simulink model "untuk_SS_closedLoop"  (R2021b)
settings: Solver=VariableStepAuto  StartTime=0.0  StopTime=1680  RelTol=1e-3
undefined symbols (not defined in the file): alpha, lr_init, selectorSP, sigbuilder_block, SP
libraries: slpidlib x1
settings Model: Creator=Asus  LastModifiedBy=Asus

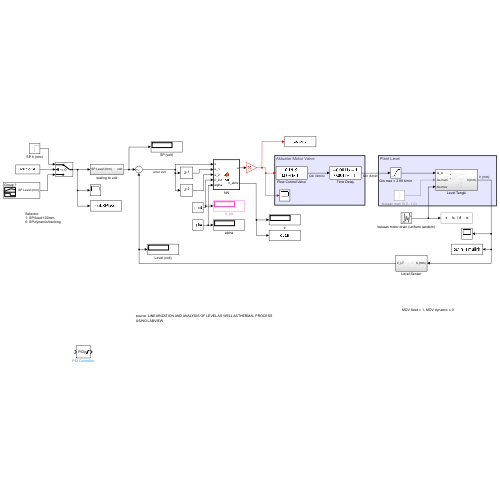
[thumbnail: Simulink's stored preview of the top-level diagram]
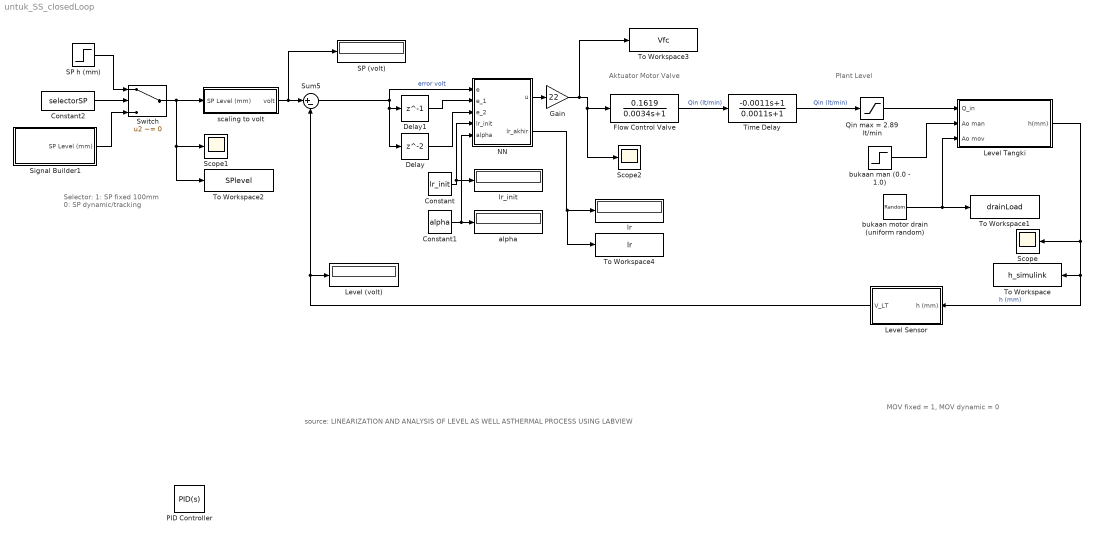
== system untuk_SS_closedLoop ==
  note: Selector:
      | 1: SP fixed 100mm
      | 0: SP dynamic/tracking
  note: Aktuator Motor Valve
  note: Plant Level
  note: source: LINEARIZATION AND ANALYSIS OF LEVEL AS WELL ASTHERMAL PROCESS USING LABVIEW
  note: MOV fixed = 1, MOV dynamic = 0
  Constant : Constant  Value=lr_init
  Constant1 : Constant  Value=alpha
  Constant2 : Constant  Value=selectorSP
  Delay : Delay  InitialCondition=0
  Delay1 : Delay  DelayLength=1  InitialCondition=0
  Flow Control Valve : TransferFcn  Numerator=[0.1619]  Denominator=[0.0034 1]
  Gain : Gain  Gain=22
  Level (volt) : Display
  Level Sensor : Subsystem
  Level Tangki : Subsystem
  NN : MATLAB Function  TreatAsAtomicUnit=on
  PID Controller : slpidlib/PID Controller  Controller=PID  Form=Parallel  TimeDomain=Continuous-time  UseExternalTs=off  SampleTime=-1  IntegratorMethod=Forward Euler  FilterMethod=Forward Euler  ControllerParametersSource=internal  P=13.8  I=0.256  D=0  UseFilter=on  N=100  TunerSelectOption=Transfer Function Based (PID Tuner App)  InitialConditionSource=internal  InitialConditionForIntegrator=0  InitialConditionForFilter=0  DifferentiatorICPrevScaledInput=0  ExternalReset=none  TrackingMode=off  Kt=1  LimitOutput=on  SatLimitsSource=internal  UpperSaturationLimit=22  LowerSaturationLimit=0  LinearizeAsGain=on  AntiWindupMode=none  Kb=1  POutMin=[]  POutMax=[]  IOutMin=[]  IOutMax=[]  DOutMin=[]  DOutMax=[]  NOutMin=[]  NOutMax=[]  SumOutMin=[]  SumOutMax=[]  SaturationOutMin=[]  SaturationOutMax=[]  PParamMin=[]  PParamMax=[]  IParamMin=[]  IParamMax=[]  DParamMin=[]  DParamMax=[]  NParamMin=[]  NParamMax=[]  KbParamMin=[]  KbParamMax=[]  KtParamMin=[]  KtParamMax=[]  KbOutMin=[]  KbOutMax=[]  KtOutMin=[]  KtOutMax=[]  IntegratorOutMin=[]  IntegratorOutMax=[]  FilterOutMin=[]  FilterOutMax=[]  SumI1OutMin=[]  SumI1OutMax=[]  SumI2OutMin=[]  SumI2OutMax=[]  SumI3OutMin=[]  SumI3OutMax=[]  SumI4OutMin=[]  SumI4OutMax=[]  SumDOutMin=[]  SumDOutMax=[]  DifferentiatorOutMin=[]  DifferentiatorOutMax=[]  FilterDiffOutCoefMin=[]  FilterDiffOutCoefMax=[]  ReciprocalOutMin=[]  ReciprocalOutMax=[]  SumDenOutMin=[]  SumDenOutMax=[]  SumNumOutMin=[]  SumNumOutMax=[]  DivideOutMin=[]  DivideOutMax=[]  UdiffTsProdOutMin=[]  UdiffTsProdOutMax=[]  NTsProdOutMin=[]  NTsProdOutMax=[]  UintegralTsProdOutMin=[]  UintegralTsProdOutMax=[]  UngainTsProdOutMin=[]  UngainTsProdOutMax=[]  IntegratorContinuousStateAttributes=''  IntegratorStateMustResolveToSignalObject=off  IntegratorRTWStateStorageClass=Auto  FilterContinuousStateAttributes=''  FilterStateMustResolveToSignalObject=off  FilterRTWStateStorageClass=Auto  ParallelPVariant=InternalParameters  IdealPVariant=Disabled  IVariant=InternalParameters  DVariant=InternalParameters  IntegratorVariant=Continuous  SatVariant=Enabled  AWVariant=Passthrough  PCopyVariant=Disabled  TRVariant=Disabled  FdbkBlocksVariant=Forward  IdealPFdbkVariant=Disabled  SatFdbkVariant=Disabled  DerivativeFilterVariant=ContFilter  NVariant=InternalParameters  NCopyVariant=Disabled  FilterICVariant=InternalICsFilter  IntegratorICVariant=InternalICs  ExternalResetVariant=Disabled  TRSumVariant=Passthrough  SumFdbkVariant=Disabled  SumVariant=Sum_PID  TsampFilterVariant=InternalTs  TsampNgainVariant=Passthrough  TsampIntegralVariant=Passthrough  ExternalSaturationOutDataTypeStr=Inherit: Same as second input
  Qin max = 2.89 lt/min : Saturate  UpperLimit=2.89254556517870  LowerLimit=0
  SP (volt) : Display
  SP h (mm) : Step  Time=0  After=SP  SampleTime=0.1
  Scope : Scope
  Scope1 : Scope
  Scope2 : Scope
  Signal Builder1 : Subsystem  Tag=STV Subsys  LoadFcn=sigbuilder_block('load');  StartFcn=sigbuilder_block('start');  StopFcn=sigbuilder_block('stop');  ClipboardFcn=sigbuilder_block('clipboard');  mask(Sigbuilder block){tuvar=[0:10]}
      mask help: Simulink:masks:SigbuilderBlock_MD
      mask init:
      | if ~strcmp(get_param(bdroot(gcbh),'SimulationStatus'),'stopped') tuvar = sigbuilder_block('maskInit'); end
      settings: CopyFcn=sigbuilder_block('copy');  DeleteFcn=sigbuilder_block('delete');  ModelCloseFcn=sigbuilder_block('modelClose');  PreSaveFcn=sigbuilder_block('preSave');  PauseFcn=sigbuilder_block('pause');  ContinueFcn=sigbuilder_block('continue');  NameChangeFcn=sigbuilder_block('namechange');  OpenFcn=sigbuilder_block('open',[572.4 148.2 550.8 400.2 ]);  CloseFcn=sigbuilder_block('close');
      mask Display: plot(0, 0, 100, 100,[2, 2, 32, 32, 2], [68, 8, 8, 68, 68],[32, 2], [38, 38], [32, 19, 2],[53, 60, 44], [32, 17, 17, 2],[16, 16, 31, 31]);txt = getActiveGroup(gcbh);text(2, 100, txt,'verticalAlignment', 'top');
  Sum5 : Sum  Inputs=|+-
  Switch : Switch  Criteria=u2 ~= 0
  Time Delay : TransferFcn  Numerator=[-0.0011 1]  Denominator=[0.0011 1]
  To Workspace : ToWorkspace  VariableName=h_simulink  SampleTime=-1
      settings: Save2DSignal=2-D array (concatenate along first dimension)
  To Workspace1 : ToWorkspace  VariableName=drainLoad  SampleTime=-1
  To Workspace2 : ToWorkspace  VariableName=SPlevel  SampleTime=-1
  To Workspace3 : ToWorkspace  VariableName=Vfc  SampleTime=-1
  To Workspace4 : ToWorkspace  VariableName=lr  SampleTime=-1
  alpha : Display
  bukaan man (0.0 - 1.0) : Step  Time=0  SampleTime=0
  bukaan motor drain (uniform random) : UniformRandomNumber  Minimum=0  SampleTime=15
  lr : Display
  lr_init : Display
  scaling to volt : Subsystem
  wires:
  Sum5/1 -> Delay/1, Delay1/1, NN/1(e)  "error volt"
  Delay1/1 -> NN/2(e_1)
  Delay/1 -> NN/3(e_2)
  Level Tangki/1(h(mm)) -> Level Sensor/1(h (mm)), To Workspace/1, Scope/1  "h (mm)"
  Qin max = 2.89 lt/min/1 -> Level Tangki/1(Q_in)
  Level Sensor/1(V_LT) -> Sum5/2, Level (volt)/1
  bukaan man (0.0 - 1.0)/1 -> Level Tangki/2(Ao man)
  bukaan motor drain (uniform random)/1 -> Level Tangki/3(Ao mov), To Workspace1/1
  scaling to volt/1(volt) -> SP (volt)/1, Sum5/1
  Switch/1 -> scaling to volt/1(SP Level (mm)), To Workspace2/1, Scope1/1
  Constant/1 -> NN/4(lr_init), lr_init/1
  Constant1/1 -> NN/5(alpha), alpha/1
  SP h (mm)/1 -> Switch/1
  Signal Builder1/1(SP Level (mm)) -> Switch/3
  Constant2/1 -> Switch/2
  NN/2(lr_akhir) -> To Workspace4/1, lr/1
  Flow Control Valve/1 -> Time Delay/1  "Qin (lt/min)"
  Time Delay/1 -> Qin max = 2.89 lt/min/1  "Qin (lt/min)"
  Gain/1 -> To Workspace3/1, Scope2/1, Flow Control Valve/1
  NN/1(u) -> Gain/1

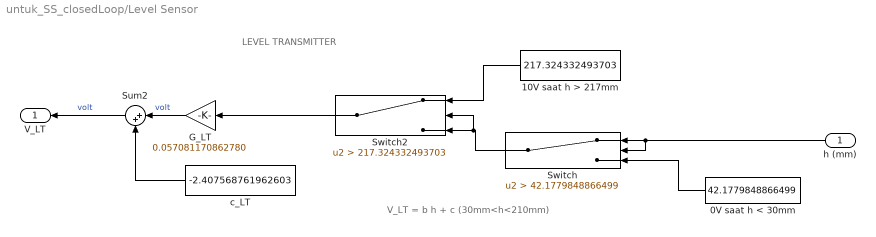
== system untuk_SS_closedLoop/Level Sensor ==
  note: V_LT = b h + c (30mm<h<210mm)
  note: LEVEL TRANSMITTER
  h (mm) : Inport
  0V saat h < 30mm : Constant  Value=42.1779848866499
  10V saat h > 217mm : Constant  Value=217.324332493703
  G_LT : Gain  Gain=0.057081170862780
  Sum2 : Sum  Inputs=|++
  Switch : Switch  Criteria=u2 > Threshold  Threshold=42.1779848866499
  Switch2 : Switch  Criteria=u2 > Threshold  Threshold=217.324332493703
  c_LT : Constant  Value=-2.407568761962603
  V_LT : Outport
  wires:
  Switch/1 -> Switch2/2, Switch2/3
  10V saat h > 217mm/1 -> Switch2/1
  G_LT/1 -> Sum2/1  "volt"
  0V saat h < 30mm/1 -> Switch/3
  c_LT/1 -> Sum2/2
  h (mm)/1 -> Switch/2, Switch/1
  Switch2/1 -> G_LT/1
  Sum2/1 -> V_LT/1  "volt"

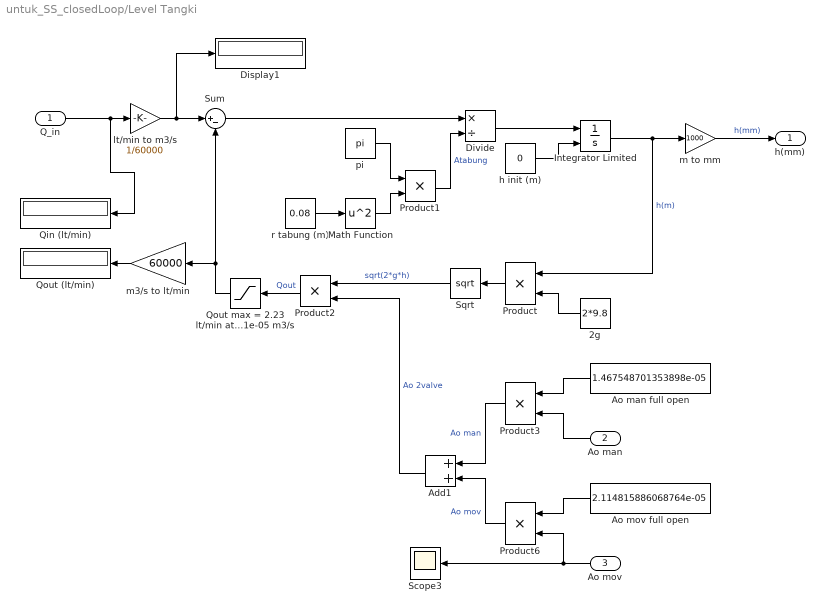
== system untuk_SS_closedLoop/Level Tangki ==
  Q_in : Inport
  Ao man : Inport  Port=2
  Ao mov : Inport  Port=3
  2g : Constant  Value=2*9.8
  Add1 : Sum
  Ao man full open : Constant  Value=1.467548701353898e-05
  Ao mov full open : Constant  Value=2.114815886068764e-05
  Display1 : Display
  Divide : Product  Inputs=*/
  Integrator Limited : Integrator  InitialConditionSource=external  LimitOutput=on  UpperSaturationLimit=1  LowerSaturationLimit=0
  Math Function : Math  Operator=square  SaturateOnIntegerOverflow=on
  Product{,1..3,6} (5 alike) : Product
  Qin (lt/min) : Display
  Qout (lt/min) : Display
  Qout max = 2.23 lt/min atau 3.716859357396591e-05 m3/s : Saturate  UpperLimit=3.716859357396591e-05  LowerLimit=0
  Scope3 : Scope
  Sqrt : Sqrt  SaturateOnIntegerOverflow=on
  Sum : Sum  Inputs=|+-
  h init (m) : Constant  Value=0
  lt/min to m3/s : Gain  Gain=1/60000
  m to mm : Gain  Gain=1000
  m3/s to lt/min : Gain  Gain=60000
  pi : Constant  Value=pi
  r tabung (m) : Constant  Value=0.08
  h(mm) : Outport
  wires:
  Sqrt/1 -> Product2/1  "sqrt(2*g*h)"
  h init (m)/1 -> Integrator Limited/2
  Sum/1 -> Divide/1
  Math Function/1 -> Product1/2
  Qout max = 2.23 lt/min atau 3.716859357396591e-05 m3/s/1 -> Sum/2, m3/s to lt/min/1
  Integrator Limited/1 -> Product/1, m to mm/1  "h(m)"
  Divide/1 -> Integrator Limited/1
  r tabung (m)/1 -> Math Function/1
  Product1/1 -> Divide/2  "Atabung"
  lt/min to m3/s/1 -> Display1/1, Sum/1
  pi/1 -> Product1/1
  Product/1 -> Sqrt/1
  m3/s to lt/min/1 -> Qout (lt/min)/1
  Q_in/1 -> Qin (lt/min)/1, lt/min to m3/s/1
  Product2/1 -> Qout max = 2.23 lt/min atau 3.716859357396591e-05 m3/s/1  "Qout"
  2g/1 -> Product/2
  m to mm/1 -> h(mm)/1  "h(mm)"
  Ao mov full open/1 -> Product6/1
  Ao man full open/1 -> Product3/1
  Product6/1 -> Add1/2  "Ao mov"
  Product3/1 -> Add1/1  "Ao man"
  Ao man/1 -> Product3/2
  Ao mov/1 -> Scope3/1, Product6/2
  Add1/1 -> Product2/2  "Ao 2valve"

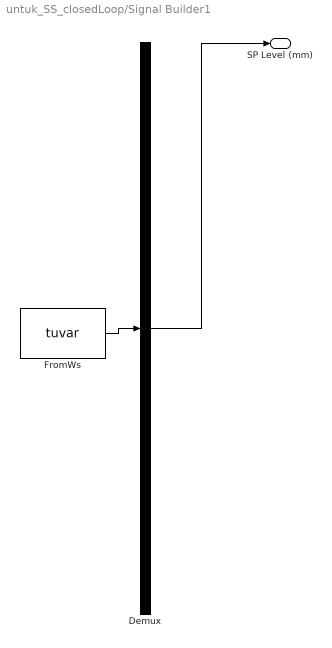
== system untuk_SS_closedLoop/Signal Builder1 ==
  Demux : Demux  Tag=STV Demux  Outputs=1
      settings: DisplayOption=none
  FromWs : FromWorkspace  Tag=STV FromWs  VariableName=tuvar
      SigBuilderData=|
      | common.afterFinalStr = 'Extrapolate'
      | common.sampleTime = 0
      | dataSet.timeRange = [0 1680]
      | dataSet.name = 'Group 1'
      | sbobj.Groups.Name = 'Group 1'
      | sbobj.Groups.Signals.Name = 'SP Level (mm)'
      | sbobj.Groups.Signals.XData = [0 240 240 480 480 720 720 960 960 1200 1200 1440 1440 1680]
      | sbobj.Groups.Signals.YData = [50 50 100 100 150 150 200 200 150 150 100 100 50 50]
      | sbobj.Groups.TimeRange = [0 1680]
  SP Level (mm) : Outport  Tag=STV Outport
  wires:
  Demux/1 -> SP Level (mm)/1
  FromWs/1 -> Demux/1

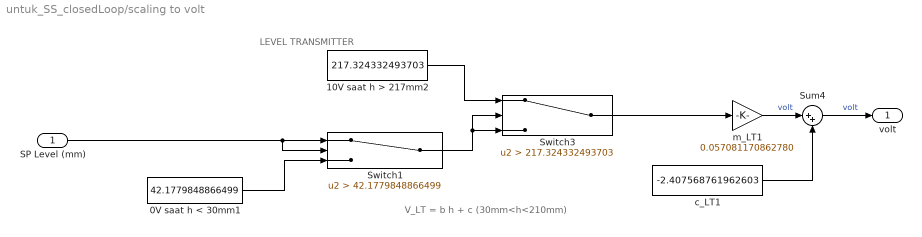
== system untuk_SS_closedLoop/scaling to volt ==
  note: LEVEL TRANSMITTER
  note: V_LT = b h + c (30mm<h<210mm)
  SP Level (mm) : Inport
  0V saat h < 30mm1 : Constant  Value=42.1779848866499
  10V saat h > 217mm2 : Constant  Value=217.324332493703
  Sum4 : Sum  Inputs=|++
  Switch1 : Switch  Criteria=u2 > Threshold  Threshold=42.1779848866499
  Switch3 : Switch  Criteria=u2 > Threshold  Threshold=217.324332493703
  c_LT1 : Constant  Value=-2.407568761962603
  m_LT1 : Gain  Gain=0.057081170862780
  volt : Outport
  wires:
  Switch1/1 -> Switch3/2, Switch3/3
  SP Level (mm)/1 -> Switch1/1, Switch1/2
  10V saat h > 217mm2/1 -> Switch3/1
  0V saat h < 30mm1/1 -> Switch1/3
  m_LT1/1 -> Sum4/1  "volt"
  Switch3/1 -> m_LT1/1
  c_LT1/1 -> Sum4/2
  Sum4/1 -> volt/1  "volt"

== matlab function untuk_SS_closedLoop/NN ==
  settings: updateMethod=DISCRETE
  data: u output; e input; e_1 input; e_2 input; lr_init input; alpha input; lr_akhir output
function [u,lr_akhir] = fcn(e, e_1, e_2, lr_init, alpha)
    % initial condition
    persistent w_input v_hidden y_hidden delta2 hj ei_1 ei_2  lr n
    persistent v_hidden2 delta2_1 hj1
    if isempty(w_input)
        w_input = rand(3,3);
        n = 0;
    end
    if isempty(v_hidden)
        v_hidden = rand(1,3);
    end
    if isempty(delta2)
        delta2 = zeros(1,3);
    end
    if isempty(hj)
        hj = [0;0;0];
        hj1 = [0;0;0];
    end
    if isempty(ei_1)
        ei_1 = 0;
    end
    if isempty(ei_2)
        ei_2 = 0;
    end
    if isempty(lr)
        lr = lr_init;
    end
    ei = e;
    x_input = [ei; ei_1; ei_2];
    % FORWARD PROPAGATION
    % Input layer to hidden layer
    for j_hiddenLayer = 1:3
        Sj = w_input(j_hiddenLayer,:) * x_input; % summing hidden neuron ke-j
        hj(j_hiddenLayer) = 1/(1 + exp(-1*Sj));
    end
    
    % hidden layer to output layer
    r = v_hidden * hj;
    u = 1/(1+exp(-1*r));

    % BACKWARD PROPAGATION: BACKPROPAGATION
    if ei <= 0.0571
        delta_lr = 0;
    else
        delta_lr = alpha*ei;
    end
    lr = lr + delta_lr;
    delta1 = ei*u*(1-u);
    dey_deu =   1;
    for j_hiddenLayer = 1:3
        v_hidden(j_hiddenLayer) = v_hidden(j_hiddenLayer) + lr * dey_deu * delta1 * hj(j_hiddenLayer);
        delta2(j_hiddenLayer) = delta1 * v_hidden(j_hiddenLayer) * hj(j_hiddenLayer) * (1 - hj(j_hiddenLayer));
        
        for i_inputLayer = 1:3
            w_input(j_hiddenLayer,i_inputLayer) = w_input(j_hiddenLayer,i_inputLayer) + lr * dey_deu * delta2(j_hiddenLayer) * x_input(i_inputLayer);
        end
    end
    % updating variable
    ei_2 = ei_1;
    ei_1 = ei;
    w_input;
    v_hidden;
    n = n + 1;
    lr_akhir = lr;
